simulink model "RC_BALDOSA"  (R2022a)
settings: Solver=VariableStepAuto  StartTime=0.0  StopTime=60  RelTol=1e-3
settings Model: Creator=mariodelossantos  LastModifiedBy=mariodelossantos

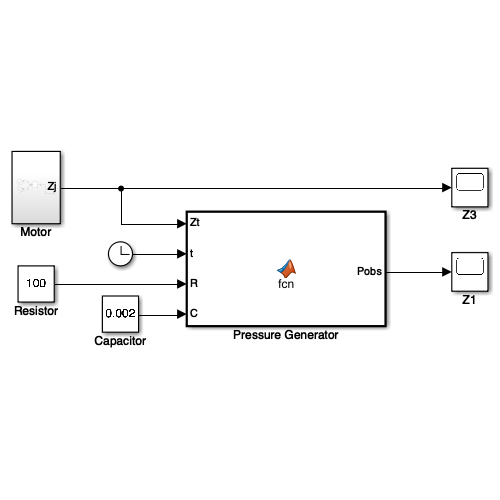
[thumbnail: Simulink's stored preview of the top-level diagram]
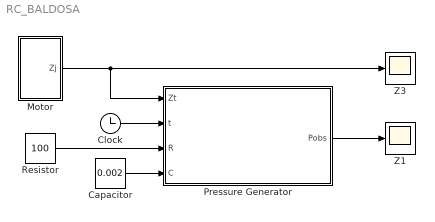
== system RC_BALDOSA ==
  Capacitor : Constant  Value=0.002
  Clock : Clock
  Motor : Subsystem
  Pressure Generator : MATLAB Function  TreatAsAtomicUnit=on
  Resistor : Constant  Value=100
  Z1 : Scope
  Z3 : Scope
  wires:
  Pressure Generator/1(Pobs) -> Z1/1
  Clock/1 -> Pressure Generator/2(t)
  Resistor/1 -> Pressure Generator/3(R)
  Capacitor/1 -> Pressure Generator/4(C)
  Motor/1(Zj) -> Pressure Generator/1(Zt), Z3/1

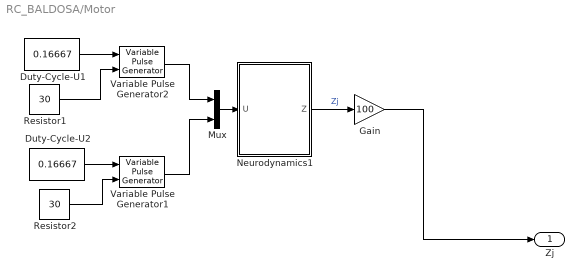
== system RC_BALDOSA/Motor ==
  Duty-Cycle-U1 : Constant  Value=0.16667  OutMin=[0]  OutMax=[0.8]
  Duty-Cycle-U2 : Constant  Value=0.16667  OutMin=[0]  OutMax=[0.8]
  Gain : Gain  Gain=100
  Mux : Mux  Inputs=2
  Neurodynamics1 : Subsystem
  Resistor1 : Constant  Value=30
  Resistor2 : Constant  Value=30
  Variable Pulse Generator1 : VariablePulseGenerator  RunAtFixedTimeIntervals=on  SampleTime=1/10.4
  Variable Pulse Generator2 : VariablePulseGenerator  RunAtFixedTimeIntervals=on  SampleTime=1/10.4
  Zj : Outport
  wires:
  Resistor1/1 -> Variable Pulse Generator2/2
  Resistor2/1 -> Variable Pulse Generator1/2
  Duty-Cycle-U2/1 -> Variable Pulse Generator1/1
  Variable Pulse Generator2/1 -> Mux/1
  Neurodynamics1/1(Z) -> Gain/1  "Zj"
  Mux/1 -> Neurodynamics1/1(U)
  Duty-Cycle-U1/1 -> Variable Pulse Generator2/1
  Variable Pulse Generator1/1 -> Mux/2
  Gain/1 -> Zj/1

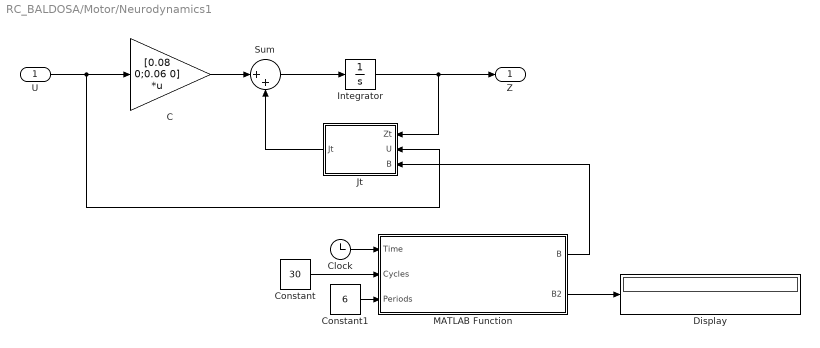
== system RC_BALDOSA/Motor/Neurodynamics1 ==
  U : Inport
  C : Gain  Gain=[0.08 0;0.06 0]  Multiplication=Matrix(K*u)
  Clock : Clock
  Constant : Constant  Value=30
  Constant1 : Constant  Value=6
  Display : Display
  Integrator : Integrator
  Jt : MATLAB Function  TreatAsAtomicUnit=on
  MATLAB Function : MATLAB Function  TreatAsAtomicUnit=on
  Sum : Sum  Inputs=|++
  Z : Outport
  wires:
  Integrator/1 -> Z/1, Jt/1(Zt)
  C/1 -> Sum/1
  Jt/1(Jt) -> Sum/2
  U/1 -> C/1, Jt/2(U)
  Sum/1 -> Integrator/1
  Constant1/1 -> MATLAB Function/3(Periods)
  Clock/1 -> MATLAB Function/1(Time)
  Constant/1 -> MATLAB Function/2(Cycles)
  MATLAB Function/2(B2) -> Display/1
  MATLAB Function/1(B) -> Jt/3(B)

== matlab function RC_BALDOSA/Pressure Generator ==
  data: Zt input; Pobs output; t input; R input; C input
function Pobs = fcn(Zt, t, R, C)

    V= Zt(1); %Voltage or system reference;
    Vc = V * (1 - exp(-t/(R*C))); % Voltage at the capacitor  
    
Pobs = Vc;

== matlab function RC_BALDOSA/Motor/Neurodynamics1/MATLAB Function ==
  settings: updateMethod=DISCRETE
  data: Time input; B output; Cycles input; Periods input; B2 output
function [B, B2] = ControlledDynamic_B(Time, Cycles, Periods)

   B = zeros(2,2,2);
   %B1 = [0 0; 0 0]; %There must be a B per stimulus
   %B2_3
   %B2 = [-0.67 -0.91 ;-0.3 -1.21];
   %B2_2
   %B2 = [-0.08 -1.08; 1.2054 -0.0076];
   %B2_1
   %B2 = [-0.02 -0.07; 0.33 -1.31];
   PCycles = zeros(6,1);
   for i = 1:Periods
       PCycles(i) = i * Cycles;   
   end
   %random_selector = randi([1,3]);

   if(Time >= 0 && Time <= PCycles(2))
%       random_selector = randi([1,3]);
%       if(random_selector == 1)
          B1 = [0 0; 0 0];
          B2 = [-0.02 -0.07; 0.33 -1.31]; 
%       elseif(random_selector == 2)
%           B1 = [0 0; 0 0];
%           B2 = [-0.08 -1.08; 1.2054 -0.0076];
%       else
%           B1 = [0 0; 0 0];
%           B2 = [-0.67 -0.91; 0.3 -1.21];
      B(:,:,1) = B1;
      B(:,:,2) = B2;
   elseif(Time >= PCycles(2)+1 && Time <= PCycles(4))
       B1 = [0 0;0 0];
       B2 = [-0.08 -1.08; 1.2054 -0.0076];
       B(:,:,1) = B1;
       B(:,:,2) = B2;
   else
       B1 = [0 0; 0 0];
       B2 = [-0.67 -0.91; -0.3 -1.21];
       B(:,:,1) = B1;
       B(:,:,2) = B2;
   end

== matlab function RC_BALDOSA/Motor/Neurodynamics1/Jt ==
  data: Zt input; U input; Jt output; B input
function Jt = fcn(Zt, U,B)
   A = [-0.16 -0.49;-0.02 -0.33];
   nRegions  = size(A,1);
   M = size(U,1); %nStimuli
   simulationLength = size(U,2);
%    B = zeros(2,2,2);
%    B1 = [0 0; 0 0]; %There must be a B per stimulus
%    %B2_3
%    B2 = [-0.67 -0.91 ;-0.3 -1.21];
%    %B2_2
%    %B2 = [-0.08 -1.08; 1.2054 -0.0076];
%    %B2_1
%    %B2 = [-0.02 -0.07; 0.33 -1.31];
%    B(:,:,1) = B1;
%    B(:,:,2) = B2;
      assert(M == size(B,3),...
       'Unexpected number of induced connectivity parameters B.');
   T = zeros(nRegions); %nRegions x nRegions
    for t = 1:simulationLength
           for uu = 1:M % Sum (Uj * Bj)
               tmp = U(uu,t)*B(:,:,uu);
               T = -0.5*exp(T + tmp);  
           end
    end
    SI = diag(A);
    A =  A - diag(exp(SI) + (SI));
Jt = (A*Zt) + (T*Zt);
